simulink model "lab1"  (R2023a)
settings: Solver=VariableStepAuto  StartTime=0.0  StopTime=10  MaxStep=0.002  RelTol=1e-5
undefined symbols (not defined in the file or in its folder): beta, C_m, C_w, J, L_a, L_o, R
settings Model: Creator=lizar  LastModifiedBy=diontep

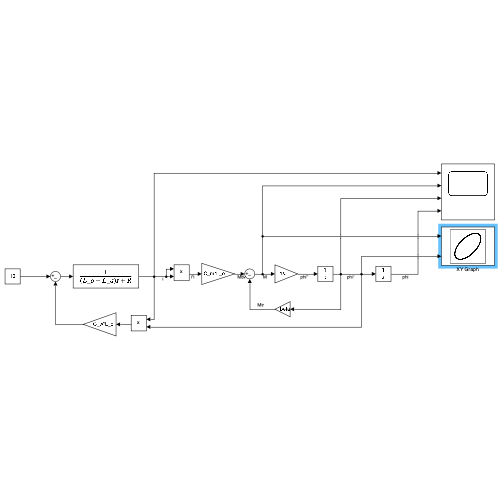
[thumbnail: Simulink's stored preview of the top-level diagram]
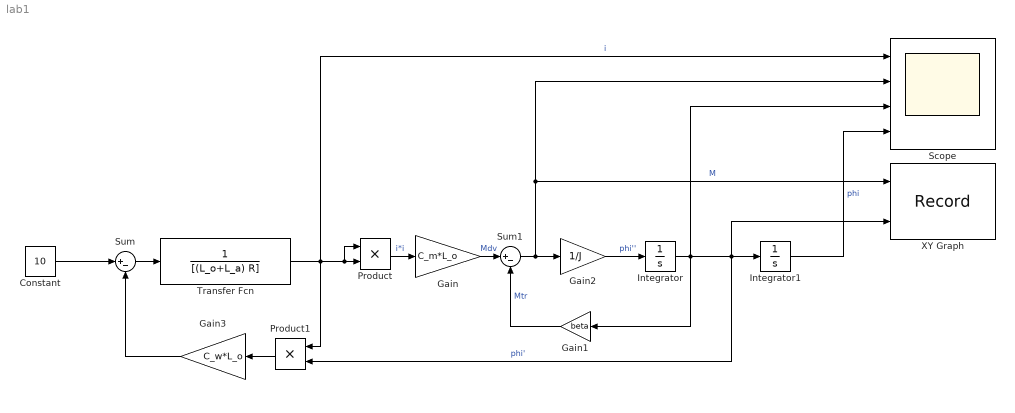
== system lab1 ==
  Constant : Constant  Value=10
  Gain : Gain  Gain=C_m*L_o
  Gain1 : Gain  Gain=beta
  Gain2 : Gain  Gain=1/J
  Gain3 : Gain  Gain=C_w*L_o
  Integrator : Integrator
  Integrator1 : Integrator
  Product : Product
  Product1 : Product
  Scope : Scope  NumInputPorts=4
  Sum : Sum  Inputs=|+-
  Sum1 : Sum  Inputs=|+-
  Transfer Fcn : TransferFcn  Denominator=[(L_o+L_a) R]
  XY Graph : Record  FileSettingsInternal="{\"entries\":[{\"content\":{\"excelSettings\":{\"content\":{},\"type\":\"Streamout.ExcelSettings\"}},\"type\":\"Streamout.FileSettingStorage\",\"uuid\":\"\"}],\"packageUris\":[\"http:\\/\\/schema.mathworks.com\\/mf0\\/streamout_blocks\\/R2020a\"],\"version\":\"1.0\"}"  Layout=[1 1]  SignalsInternal="{\"entries\":[{\"content\":{\"signals\":[{\"content\":{\"blockPath\":[],\"dimensions\":[1],\"domain\":\"\",\"lineColor\":\"#0072bd\",\"plots\":[1],\"port\":1,\"sid\":[\"\"],\"signalID\":233,\"signalName\":\"M\"},\"type\":\"RecordBlkView.Signal\",\"uuid\":\"\"},{\"content\":{\"blockPath\":[],\"dimensions\":[1],\"domain\":\"\",\"lineColor\":\"#d95319\",\"plots\":[1],\"port\":2,\"sid\":[\"\"],\"signalID\":237,\"signalName\":\"phi'\"},\"type\":\"RecordBlkView.Signal\",\"uuid\":\"\"}]},\"type\":\"RecordBlkView.InputSignals\",\"uuid\":\"\"}],\"packageUris\":[\"http:\\/\\/schema.mathworks.com\\/mf0\\/streamout_blocks\\/R2020a\"],\"version\":\"1.0\"}"  VisualizationBindings="{\"xyplotplugin\":{\"info\":[{\"series\":[{\"bindingParametersList\":[{\"parameter\":\"Y-Axis\",\"signalID\":233,\"signalName\":\"M\"},{\"parameter\":\"X-Axis\",\"signalID\":237,\"signalName\":\"phi'\"}],\"seriesID\":1310},{\"bindingParametersList\":[{\"parameter\":\"X-Axis\",\"signalID\":233,\"signalName\":\"M\"}],\"seriesID\":480}],\"subplotID\":1}]}}"  CompatibilityTag=XY
  wires:
  Integrator/1 -> Gain1/1, XY Graph/2, Product1/2, Integrator1/1, Scope/3  "phi'"
  Sum/1 -> Transfer Fcn/1
  Transfer Fcn/1 -> Scope/1, Product/1, Product/2, Product1/1  "i"
  Product/1 -> Gain/1  "i*i"
  Sum1/1 -> Gain2/1, Scope/2, XY Graph/1  "M"
  Product1/1 -> Gain3/1
  Gain2/1 -> Integrator/1  "phi''"
  Gain3/1 -> Sum/2
  Constant/1 -> Sum/1
  Integrator1/1 -> Scope/4  "phi"
  Gain/1 -> Sum1/1  "Mdv"
  Gain1/1 -> Sum1/2  "Mtr"
